simulink model "untitled"  (R2023b)
settings: Solver=VariableStepAuto  StartTime=0.0  StopTime=10^6  RelTol=1e-3
settings Model: Creator=kBen  LastModifiedBy=kBen

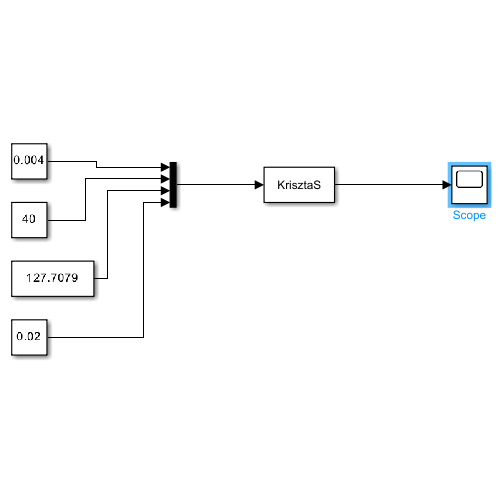
[thumbnail: Simulink's stored preview of the top-level diagram]
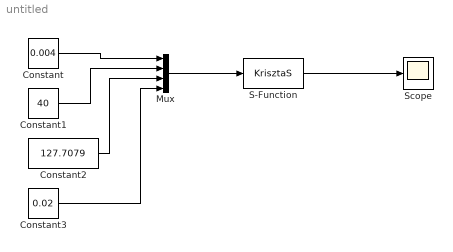
== system untitled ==
  Constant : Constant  Value=0.004
  Constant1 : Constant  Value=40
  Constant2 : Constant  Value=127.7079
  Constant3 : Constant  Value=0.02
  Mux : Mux
  S-Function : S-Function  FunctionName=KrisztaS  SFunctionDeploymentMode=off  EnableBusSupport=off
  Scope : Scope
  wires:
  Mux/1 -> S-Function/1
  S-Function/1 -> Scope/1
  Constant/1 -> Mux/1
  Constant1/1 -> Mux/2
  Constant2/1 -> Mux/3
  Constant3/1 -> Mux/4
